simulink model "InvertedPend_Full_state"  (R2016b)
settings: Solver=ode45  StartTime=0.0  StopTime=12  MaxStep=1e-3  RelTol=1e-3  EnableMultiTasking=on
values from neighbouring files (symbols this model uses):
  J = 0.5*(M)*(r)^2    (= 1.404536e-05)    [constants.m]
  K1 = [-1.15729318091470,-0.0495037685039268,-0.228035085025578,-0.244895733178026]    [pendulum.m]
  L = (120/1000)    (= 0.12)    [constants.m]
  m = 0.550    (= 0.55)    [constants.m]
  N_bar = -inv(Cn*((A-B*K1)\B))    [pendulum.m]
  r = 0.028    [constants.m]
undefined symbols (not defined in the file): M
settings Model: Creator=Patrick  LastModifiedBy=Craig
settings DataIOCC: LimitDataPoints=on  SaveFormat=Array  SignalLoggingSaveFormat=ModelDataLogs
settings OptimizationCC: ExpressionDepthLimit=2147483647  LifeSpan=inf
settings DebuggingCC: UnderspecifiedInitializationDetection=Classic  MergeDetectMultiDrivingBlocksExec=none  SolverPrmCheckMsg=warning  FcnCallInpInsideContextMsg=warning  StateNameClashWarn=warning  SFUnexpectedBacktrackingDiag=warning  SFNoUnconditionalDefaultTransitionDiag=warning  SFExecutionAtInitializationDiag=none
settings HardwareCC: ProdBitPerPointer=32  ProdBitPerSizeT=32  ProdBitPerPtrDiffT=32  ProdLargestAtomicFloat=None  ProdIntDivRoundTo=Undefined  ProdEndianess=Unspecified  ProdWordSize=32  ProdHWDeviceType=32-bit Generic
settings ModelReferenceCC: PropagateSignalLabelsOutOfModel=off
settings GRTTargetCC: TargetLangStandard=C89/C90 (ANSI)  GeneratePreprocessorConditionals=Disable all  CombineOutputUpdateFcns=off  GRTInterface=on
settings ConfigComp: CovMetricSettings=dw  CovHtmlReporting=on  CovSaveCumulativeToWorkspaceVar=on  CovSaveSingleToWorkspaceVar=on  CovExternalEMLEnable=off

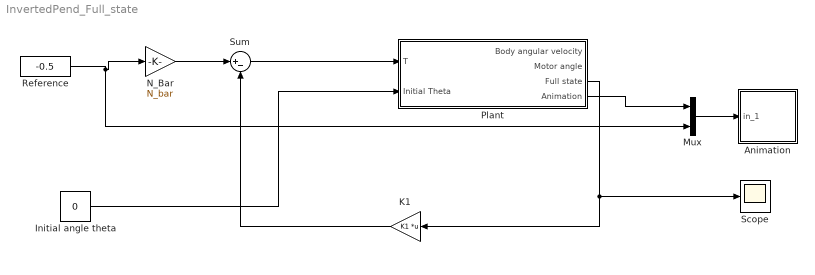
== system InvertedPend_Full_state ==
  Animation : Subsystem  mask(Pendulum plot){RefBlock=Reference, L=L, r=r, Ts=1e-3}
      mask prompts: RefBlock "DC reference signal block name:"; L "Location of mass"; r "Radius of wheel"; Ts "Simulation time step"
      mask help: Pendulum plot
      mask Help: Pendulum animation function using Handle graphics.
      mask Display: plot([-10 10],[0 0],[-2 -2 2 2],[0 1 1 0],[0 3],[1 5])
  "Initial angle theta " : Constant  Value=0
  K1 : Gain  Gain=K1  Multiplication=Matrix(K*u)
  Mux : Mux  Inputs=2
  "N_Bar " : Gain  Gain=N_bar
  Plant : Subsystem  mask{m=m, mw=M, J=J, r=r, L=L, g=9.81, theta0=0.1}
      mask prompts: m "Mass of body"; mw "Mass of wheel"; J "Inertia of wheel"; r "Radius of wheel"; L "Height of body COM"; g "Gravity"; theta0 "Initial angle"
  Reference : Constant  Value=-0.5
  Scope : Scope
  Sum : Sum  Inputs=|+-
  wires:
  Mux/1 -> Animation/1(in_1)
  Plant/4(Animation) -> Mux/1
  Sum/1 -> Plant/1(T)
  K1/1 -> Sum/2
  Plant/3(Full state) -> K1/1, Scope/1
  Reference/1 -> "N_Bar "/1, Mux/2
  "Initial angle theta "/1 -> Plant/2(Initial Theta)
  "N_Bar "/1 -> Sum/1

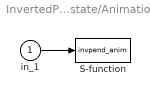
== system InvertedPend_Full_state/Animation ==
  in_1 : Inport
  S-function : S-Function  FunctionName=invpend_anim  Parameters=RefBlock,L,r,Ts  SFunctionDeploymentMode=off  EnableBusSupport=off
      settings: DeleteFcn=pendan([],[],[],'DeleteBlock');
  wires:
  in_1/1 -> S-function/1

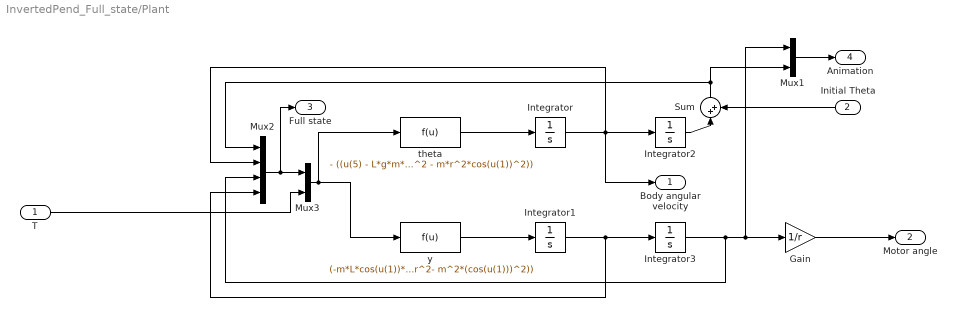
== system InvertedPend_Full_state/Plant ==
  T : Inport
  Initial Theta : Inport  Port=2
  Gain : Gain  Gain=1/r
  Integrator{,1..3} (4 alike) : Integrator
  Mux1 : Mux  Inputs=2
  Mux2 : Mux
  Mux3 : Mux  Inputs=2
  Sum : Sum  Inputs=|++
  theta : Fcn  Expr=- ((u(5) - L*g*m*sin(u(1)))*(J + m*r^2 + mw*r^2))/(L^2*m*(J + m*r^2 + mw*r^2 - m*r^2*cos(u(1))^2)) - (r^2*cos(u(1))*(u(5)/r + L*m*u(2)^2*sin(u(1))))/(L*(J + m*r^2 + mw*r^2 - m*r^2*cos(u(1))^2))
  y : Fcn  Expr=(-m*L*cos(u(1))*(m*g*L*sin(u(1)) - u(5)) + m*L^2*(m*L*u(2)^2*sin(u(1))+u(5)/r))/(L^2*(m^2+m*mw+(m*J)/r^2- m^2*(cos(u(1)))^2))
  Body angular velocity : Outport
  Motor angle : Outport  Port=2
  Full state : Outport  Port=3
  Animation : Outport  Port=4
  wires:
  y/1 -> Integrator1/1
  Integrator/1 -> Body angular velocity/1, Integrator2/1, Mux2/2
  Integrator1/1 -> Integrator3/1, Mux2/4
  Integrator3/1 -> Gain/1, Mux1/1, Mux2/3
  T/1 -> Mux3/2
  Gain/1 -> Motor angle/1
  Integrator2/1 -> Sum/1
  Sum/1 -> Mux1/2, Mux2/1
  Initial Theta/1 -> Sum/2
  Mux1/1 -> Animation/1
  Mux2/1 -> Mux3/1, Full state/1
  Mux3/1 -> theta/1, y/1
  theta/1 -> Integrator/1
